simulink model "test_derivative"  (R2024a)
settings: Solver=ode1  StartTime=0.0  StopTime=71.805  FixedStep=STEP_SIZE  RelTol=1e-3
libraries: simulink x1
settings Model: Creator=Huan  LastModifiedBy=Huan

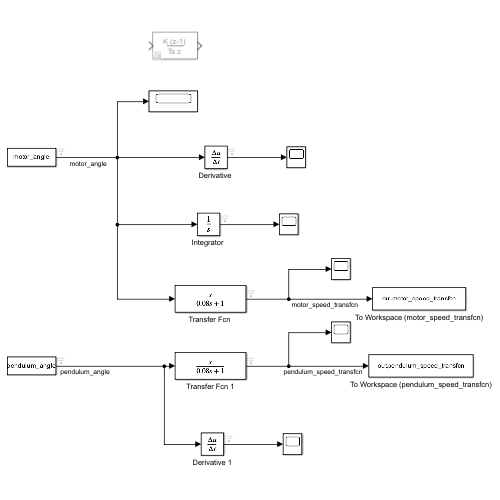
[thumbnail: Simulink's stored preview of the top-level diagram]
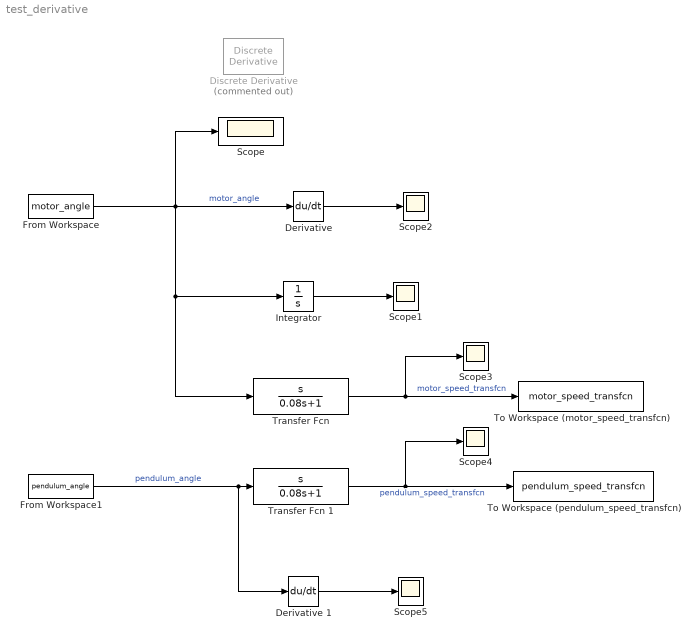
== system test_derivative ==
  "Derivative " : Derivative
  Derivative 1 : Derivative
  Discrete Derivative : simulink/Discrete/Discrete Derivative  Commented=on  gainval=1.0  ICPrevScaledInput=0.0  OutMin=[]  OutMax=[]  OutDataType=fixdt(1, 16)  OutScaling=2^-10  DoSatur=off
  From Workspace : FromWorkspace  VariableName=motor_angle  SampleTime=-1
  From Workspace1 : FromWorkspace  VariableName=pendulum_angle  SampleTime=-1
  "Integrator " : Integrator
  Scope{,1..5} (6 alike) : Scope
  To Workspace (motor_speed_transfcn) : ToWorkspace  VariableName=motor_speed_transfcn  SaveFormat=Timeseries  SampleTime=-1
  To Workspace (pendulum_speed_transfcn) : ToWorkspace  VariableName=pendulum_speed_transfcn  SaveFormat=Timeseries  SampleTime=-1
  "Transfer Fcn " : TransferFcn  Numerator=[1 0]  Denominator=[0.08 1]
  Transfer Fcn 1 : TransferFcn  Numerator=[1 0]  Denominator=[0.08 1]
  wires:
  "Integrator "/1 -> Scope1/1
  "Derivative "/1 -> Scope2/1
  "Transfer Fcn "/1 -> Scope3/1, To Workspace (motor_speed_transfcn)/1  "motor_speed_transfcn"
  From Workspace/1 -> Scope/1, "Derivative "/1, "Transfer Fcn "/1, "Integrator "/1  "motor_angle"
  Transfer Fcn 1/1 -> To Workspace (pendulum_speed_transfcn)/1, Scope4/1  "pendulum_speed_transfcn"
  From Workspace1/1 -> Derivative 1/1, Transfer Fcn 1/1  "pendulum_angle"
  Derivative 1/1 -> Scope5/1
